simulink model "cruise"  (R2021a)
settings: Solver=VariableStepAuto  StartTime=0.0  StopTime=150.0  RelTol=1e-3
model workspace (MAT data in the model file):
  aeroCoeff.Cl0 = 0
  aeroCoeff.Cl_beta = -0.051919818
  aeroCoeff.Cl_da = -0.0981676066
  aeroCoeff.Cl_dr = 0.1746396276
  aeroCoeff.Cl_p = -0.7461562431
  aeroCoeff.Cl_r = 0.1584677463
  aeroCoeff.Cm0 = 0
  aeroCoeff.Cm_alpha = -0.208453958
  aeroCoeff.Cm_de = -3.8146754263
  aeroCoeff.Cm_q = -22.9669011845
  aeroCoeff.Cn0 = 0
  aeroCoeff.Cn_beta = 0.0540377505
  aeroCoeff.Cn_beta_dot = 0
  aeroCoeff.Cn_da = 0.0101277353
  aeroCoeff.Cn_dr = -0.4423152173
  aeroCoeff.Cn_p = -0.0208253137
  aeroCoeff.Cn_r = -0.0816662365
  aeroCoeff.Cx0 = 0
  aeroCoeff.Cx_alpha = 0.2466037589
  aeroCoeff.Cx_q = 0
  aeroCoeff.Cx_de = 0
  aeroCoeff.Cy0 = 0
  aeroCoeff.Cy_beta = -0.1443361205
  aeroCoeff.Cy_beta_dot = 0
  aeroCoeff.Cy_da = 0
  aeroCoeff.Cy_dr = 0.8693004869
  aeroCoeff.Cy_p = -0.0224336303
  aeroCoeff.Cy_r = 0.1468814604
  aeroCoeff.Cz0 = -0.5167063636
  aeroCoeff.Cz_alpha = -3.6783451837
  aeroCoeff.Cz_de = 0
  aeroCoeff.Cz_q = 2.429400573
  aeroCoeff.Cx_u = -0.1637449639
  aeroCoeff.Cz_u = -0.0248990234
  aeroCoeff.Cm_u = 0.0061871085
  aeroCoeff.Cx_alpha_dot = 0
  aeroCoeff.Cz_alpha_dot = -3.5068180832
  aeroCoeff.Cm_alpha_dot = -9.6904377913
  aeroCoeff.CL = 0.515838963283
  asymmSys.P = [-3.42306054866  0  0  0; 0  -0.05686151405  0  0; 0  0  -0.306843147582  0.0431305629131; 0  0  0.0431305629131  -1.21984185712]
  asymmSys.Q = [0.1443361205  -0.515838963283  0.0224336303  60.0530728646; 0  0  -1  0; 0.051919818  0  0.7461562431  -0.1584677463; -0.0540377505  0  0.0208253137  0.0816662365]
  asymmSys.R = [0  -0.8693004869; 0  0; 0.0981676066  -0.1746396276; -0.0101277353  0.4423152173]
  asymmSys.A = [-0.0421658099377  0.150695249456  -0.0065536761565  -17.5436782408; 0  0  17.5865876368  0; -0.163793657992  0  -2.44627629671  0.509567569731; 0.0385076455239  0  -0.103566365329  -0.0489311790925]
  asymmSys.B = [0  0.253954166029; 0  0; -0.32035276129  0.520769765047; -0.00302437533493  -0.344187340133]
  g = 9.80665
  initCond.x0 = [0 0 -1000]
  initCond.v0 = 72.1867618534
  initCond.euler0 = [0 0 0]
  initCond.w0 = [0 0 0]
  rho = 1.11164
  symmSys.P = [-3.42306054866  0  0  0; 0  -3.48452116909  0  0; 0  0  -0.0175260361321  0; 0  -0.169834962866  0  -14.0221567703]
  symmSys.Q = [0.1637449639  -0.2466037589  0.5167063636  0; 0.0248990234  3.6783451837  0  -197.742278103; 0  0  0  -1; -0.0061871085  0.208453958  0  22.9669011845]
  symmSys.R = [0; 0; 0; 3.8146754263]
  symmSys.A = [-0.047835836256  0.072041892159  -0.150948648514  0; -0.00714560830362  -1.05562428959  0  56.7487664754; 0  0  0  57.0579674984; 0.000527784900863  -0.00208042503405  0  -2.32523615059]
  symmSys.B = [0; 0; 0; -0.272046268544]
  vehicle.Sref = 19.8213410712
  vehicle.cbar = 1.2651477965
  vehicle.bref = 8.2092971467
  vehicle.Ixx = 8223.41527293
  vehicle.Iyy = 17849.353945
  vehicle.Izz = 32689.1284826
  vehicle.Ixz = 1155.55423289
  vehicle.m = 2722.32108207
  vehicle.Kxx = 0.04482
  vehicle.Kyy = 4.09638
  vehicle.Kzz = 0.17818
  vehicle.Kxz = 0.0063
  vehicle.mu_c = 97.6564387652
  vehicle.mu_b = 15.0499885812
  vehicle.aileron_max = 0.523598775598
  vehicle.aileron_min = -0.523598775598
  vehicle.elevator_max = 0.305432619099
  vehicle.elevator_min = -0.305432619099
  vehicle.rudder_max = 0.436332312999
  vehicle.rudder_min = -0.436332312999
libraries: pid_lib x4
settings Model: OrderedModelArguments=off  Creator=jakob  LastModifiedBy=jakob

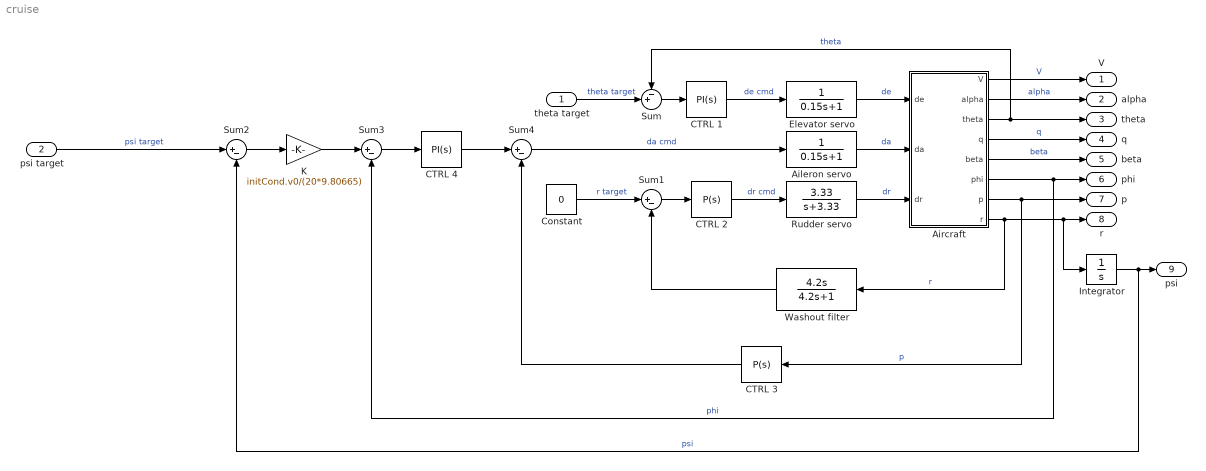
== system cruise ==
  theta target : Inport
  psi target : Inport  Port=2
  Aileron servo : TransferFcn  Denominator=[0.15 1]
  Aircraft : Subsystem
  CTRL 1 : pid_lib/PID Controller  Controller=PI  Form=Parallel  TimeDomain=Continuous-time  UseExternalTs=off  SampleTime=-1  IntegratorMethod=Forward Euler  FilterMethod=Forward Euler  ControllerParametersSource=internal  P=-0.0959107161615802  I=-0.00101116230830857  D=0  UseFilter=on  N=100  TunerSelectOption=Transfer Function Based (PID Tuner App)  InitialConditionSource=internal  InitialConditionForIntegrator=0  InitialConditionForFilter=0  DifferentiatorICPrevScaledInput=0  ExternalReset=none  TrackingMode=off  Kt=1  LimitOutput=off  SatLimitsSource=internal  UpperSaturationLimit=inf  LowerSaturationLimit=-inf  LinearizeAsGain=on  AntiWindupMode=none  Kb=1  POutMin=[]  POutMax=[]  IOutMin=[]  IOutMax=[]  DOutMin=[]  DOutMax=[]  NOutMin=[]  NOutMax=[]  SumOutMin=[]  SumOutMax=[]  SaturationOutMin=[]  SaturationOutMax=[]  PParamMin=[]  PParamMax=[]  IParamMin=[]  IParamMax=[]  DParamMin=[]  DParamMax=[]  NParamMin=[]  NParamMax=[]  KbParamMin=[]  KbParamMax=[]  KtParamMin=[]  KtParamMax=[]  KbOutMin=[]  KbOutMax=[]  KtOutMin=[]  KtOutMax=[]  IntegratorOutMin=[]  IntegratorOutMax=[]  FilterOutMin=[]  FilterOutMax=[]  SumI1OutMin=[]  SumI1OutMax=[]  SumI2OutMin=[]  SumI2OutMax=[]  SumI3OutMin=[]  SumI3OutMax=[]  SumI4OutMin=[]  SumI4OutMax=[]  SumDOutMin=[]  SumDOutMax=[]  DifferentiatorOutMin=[]  DifferentiatorOutMax=[]  FilterDiffOutCoefMin=[]  FilterDiffOutCoefMax=[]  ReciprocalOutMin=[]  ReciprocalOutMax=[]  SumDenOutMin=[]  SumDenOutMax=[]  SumNumOutMin=[]  SumNumOutMax=[]  DivideOutMin=[]  DivideOutMax=[]  UdiffTsProdOutMin=[]  UdiffTsProdOutMax=[]  NTsProdOutMin=[]  NTsProdOutMax=[]  UintegralTsProdOutMin=[]  UintegralTsProdOutMax=[]  UngainTsProdOutMin=[]  UngainTsProdOutMax=[]  IntegratorContinuousStateAttributes=''  IntegratorStateMustResolveToSignalObject=off  IntegratorRTWStateStorageClass=Auto  FilterContinuousStateAttributes=''  FilterStateMustResolveToSignalObject=off  FilterRTWStateStorageClass=Auto  ParallelPVariant=InternalParameters  IdealPVariant=Disabled  IVariant=InternalParameters  DVariant=Disabled  IntegratorVariant=Continuous  SatVariant=Disabled  AWVariant=Passthrough  PCopyVariant=Disabled  TRVariant=Disabled  FdbkBlocksVariant=Forward  IdealPFdbkVariant=Disabled  SatFdbkVariant=Disabled  DerivativeFilterVariant=Disabled  NVariant=Disabled  NCopyVariant=Disabled_SignalSpec  FilterICVariant=Disabled  IntegratorICVariant=InternalICs  ExternalResetVariant=Disabled  TRSumVariant=Passthrough  SumFdbkVariant=Disabled  SumVariant=Sum_PI  TsampFilterVariant=InternalTs  TsampNgainVariant=Passthrough  TsampIntegralVariant=Passthrough  ExternalSaturationOutDataTypeStr=Inherit: Same as second input
  CTRL 2 : pid_lib/PID Controller  Controller=P  Form=Parallel  TimeDomain=Continuous-time  UseExternalTs=off  SampleTime=-1  IntegratorMethod=Forward Euler  FilterMethod=Forward Euler  ControllerParametersSource=internal  P=-0.825543813143841  I=-0.00482340740092861  D=0  UseFilter=on  N=100  TunerSelectOption=Transfer Function Based (PID Tuner App)  InitialConditionSource=internal  InitialConditionForIntegrator=0  InitialConditionForFilter=0  DifferentiatorICPrevScaledInput=0  ExternalReset=none  TrackingMode=off  Kt=1  LimitOutput=off  SatLimitsSource=internal  UpperSaturationLimit=inf  LowerSaturationLimit=-inf  LinearizeAsGain=on  AntiWindupMode=none  Kb=1  POutMin=[]  POutMax=[]  IOutMin=[]  IOutMax=[]  DOutMin=[]  DOutMax=[]  NOutMin=[]  NOutMax=[]  SumOutMin=[]  SumOutMax=[]  SaturationOutMin=[]  SaturationOutMax=[]  PParamMin=[]  PParamMax=[]  IParamMin=[]  IParamMax=[]  DParamMin=[]  DParamMax=[]  NParamMin=[]  NParamMax=[]  KbParamMin=[]  KbParamMax=[]  KtParamMin=[]  KtParamMax=[]  KbOutMin=[]  KbOutMax=[]  KtOutMin=[]  KtOutMax=[]  IntegratorOutMin=[]  IntegratorOutMax=[]  FilterOutMin=[]  FilterOutMax=[]  SumI1OutMin=[]  SumI1OutMax=[]  SumI2OutMin=[]  SumI2OutMax=[]  SumI3OutMin=[]  SumI3OutMax=[]  SumI4OutMin=[]  SumI4OutMax=[]  SumDOutMin=[]  SumDOutMax=[]  DifferentiatorOutMin=[]  DifferentiatorOutMax=[]  FilterDiffOutCoefMin=[]  FilterDiffOutCoefMax=[]  ReciprocalOutMin=[]  ReciprocalOutMax=[]  SumDenOutMin=[]  SumDenOutMax=[]  SumNumOutMin=[]  SumNumOutMax=[]  DivideOutMin=[]  DivideOutMax=[]  UdiffTsProdOutMin=[]  UdiffTsProdOutMax=[]  NTsProdOutMin=[]  NTsProdOutMax=[]  UintegralTsProdOutMin=[]  UintegralTsProdOutMax=[]  UngainTsProdOutMin=[]  UngainTsProdOutMax=[]  IntegratorContinuousStateAttributes=''  IntegratorStateMustResolveToSignalObject=off  IntegratorRTWStateStorageClass=Auto  FilterContinuousStateAttributes=''  FilterStateMustResolveToSignalObject=off  FilterRTWStateStorageClass=Auto  ParallelPVariant=InternalParameters  IdealPVariant=Disabled  IVariant=Disabled  DVariant=Disabled  IntegratorVariant=Disabled  SatVariant=Disabled  AWVariant=Disabled  PCopyVariant=Disabled  TRVariant=Disabled  FdbkBlocksVariant=Forward  IdealPFdbkVariant=Disabled  SatFdbkVariant=Disabled  DerivativeFilterVariant=Disabled  NVariant=Disabled  NCopyVariant=Disabled_SignalSpec  FilterICVariant=Disabled  IntegratorICVariant=Disabled  ExternalResetVariant=Disabled  TRSumVariant=Passthrough  SumFdbkVariant=Disabled  SumVariant=Passthrough_P  TsampFilterVariant=InternalTs  TsampNgainVariant=Passthrough  TsampIntegralVariant=Disabled_SignalSpec  ExternalSaturationOutDataTypeStr=Inherit: Same as second input
  CTRL 3 : pid_lib/PID Controller  Controller=P  Form=Parallel  TimeDomain=Continuous-time  UseExternalTs=off  SampleTime=-1  IntegratorMethod=Forward Euler  FilterMethod=Forward Euler  ControllerParametersSource=internal  P=-2.19698599187563  I=-0.736153679717553  D=0  UseFilter=on  N=100  TunerSelectOption=Transfer Function Based (PID Tuner App)  InitialConditionSource=internal  InitialConditionForIntegrator=0  InitialConditionForFilter=0  DifferentiatorICPrevScaledInput=0  ExternalReset=none  TrackingMode=off  Kt=1  LimitOutput=off  SatLimitsSource=internal  UpperSaturationLimit=inf  LowerSaturationLimit=-inf  LinearizeAsGain=on  AntiWindupMode=none  Kb=1  POutMin=[]  POutMax=[]  IOutMin=[]  IOutMax=[]  DOutMin=[]  DOutMax=[]  NOutMin=[]  NOutMax=[]  SumOutMin=[]  SumOutMax=[]  SaturationOutMin=[]  SaturationOutMax=[]  PParamMin=[]  PParamMax=[]  IParamMin=[]  IParamMax=[]  DParamMin=[]  DParamMax=[]  NParamMin=[]  NParamMax=[]  KbParamMin=[]  KbParamMax=[]  KtParamMin=[]  KtParamMax=[]  KbOutMin=[]  KbOutMax=[]  KtOutMin=[]  KtOutMax=[]  IntegratorOutMin=[]  IntegratorOutMax=[]  FilterOutMin=[]  FilterOutMax=[]  SumI1OutMin=[]  SumI1OutMax=[]  SumI2OutMin=[]  SumI2OutMax=[]  SumI3OutMin=[]  SumI3OutMax=[]  SumI4OutMin=[]  SumI4OutMax=[]  SumDOutMin=[]  SumDOutMax=[]  DifferentiatorOutMin=[]  DifferentiatorOutMax=[]  FilterDiffOutCoefMin=[]  FilterDiffOutCoefMax=[]  ReciprocalOutMin=[]  ReciprocalOutMax=[]  SumDenOutMin=[]  SumDenOutMax=[]  SumNumOutMin=[]  SumNumOutMax=[]  DivideOutMin=[]  DivideOutMax=[]  UdiffTsProdOutMin=[]  UdiffTsProdOutMax=[]  NTsProdOutMin=[]  NTsProdOutMax=[]  UintegralTsProdOutMin=[]  UintegralTsProdOutMax=[]  UngainTsProdOutMin=[]  UngainTsProdOutMax=[]  IntegratorContinuousStateAttributes=''  IntegratorStateMustResolveToSignalObject=off  IntegratorRTWStateStorageClass=Auto  FilterContinuousStateAttributes=''  FilterStateMustResolveToSignalObject=off  FilterRTWStateStorageClass=Auto  ParallelPVariant=InternalParameters  IdealPVariant=Disabled  IVariant=Disabled  DVariant=Disabled  IntegratorVariant=Disabled  SatVariant=Disabled  AWVariant=Disabled  PCopyVariant=Disabled  TRVariant=Disabled  FdbkBlocksVariant=Forward  IdealPFdbkVariant=Disabled  SatFdbkVariant=Disabled  DerivativeFilterVariant=Disabled  NVariant=Disabled  NCopyVariant=Disabled_SignalSpec  FilterICVariant=Disabled  IntegratorICVariant=Disabled  ExternalResetVariant=Disabled  TRSumVariant=Passthrough  SumFdbkVariant=Disabled  SumVariant=Passthrough_P  TsampFilterVariant=InternalTs  TsampNgainVariant=Passthrough  TsampIntegralVariant=Disabled_SignalSpec  ExternalSaturationOutDataTypeStr=Inherit: Same as second input
  CTRL 4 : pid_lib/PID Controller  Controller=PI  Form=Parallel  TimeDomain=Continuous-time  UseExternalTs=off  SampleTime=-1  IntegratorMethod=Forward Euler  FilterMethod=Forward Euler  ControllerParametersSource=internal  P=-1.66466876697902  I=-0.145963586127284  D=-0.21492256580816  UseFilter=on  N=177.754765767358  TunerSelectOption=Transfer Function Based (PID Tuner App)  InitialConditionSource=internal  InitialConditionForIntegrator=0  InitialConditionForFilter=0  DifferentiatorICPrevScaledInput=0  ExternalReset=none  TrackingMode=off  Kt=1  LimitOutput=off  SatLimitsSource=internal  UpperSaturationLimit=inf  LowerSaturationLimit=-inf  LinearizeAsGain=on  AntiWindupMode=none  Kb=1  POutMin=[]  POutMax=[]  IOutMin=[]  IOutMax=[]  DOutMin=[]  DOutMax=[]  NOutMin=[]  NOutMax=[]  SumOutMin=[]  SumOutMax=[]  SaturationOutMin=[]  SaturationOutMax=[]  PParamMin=[]  PParamMax=[]  IParamMin=[]  IParamMax=[]  DParamMin=[]  DParamMax=[]  NParamMin=[]  NParamMax=[]  KbParamMin=[]  KbParamMax=[]  KtParamMin=[]  KtParamMax=[]  KbOutMin=[]  KbOutMax=[]  KtOutMin=[]  KtOutMax=[]  IntegratorOutMin=[]  IntegratorOutMax=[]  FilterOutMin=[]  FilterOutMax=[]  SumI1OutMin=[]  SumI1OutMax=[]  SumI2OutMin=[]  SumI2OutMax=[]  SumI3OutMin=[]  SumI3OutMax=[]  SumI4OutMin=[]  SumI4OutMax=[]  SumDOutMin=[]  SumDOutMax=[]  DifferentiatorOutMin=[]  DifferentiatorOutMax=[]  FilterDiffOutCoefMin=[]  FilterDiffOutCoefMax=[]  ReciprocalOutMin=[]  ReciprocalOutMax=[]  SumDenOutMin=[]  SumDenOutMax=[]  SumNumOutMin=[]  SumNumOutMax=[]  DivideOutMin=[]  DivideOutMax=[]  UdiffTsProdOutMin=[]  UdiffTsProdOutMax=[]  NTsProdOutMin=[]  NTsProdOutMax=[]  UintegralTsProdOutMin=[]  UintegralTsProdOutMax=[]  UngainTsProdOutMin=[]  UngainTsProdOutMax=[]  IntegratorContinuousStateAttributes=''  IntegratorStateMustResolveToSignalObject=off  IntegratorRTWStateStorageClass=Auto  FilterContinuousStateAttributes=''  FilterStateMustResolveToSignalObject=off  FilterRTWStateStorageClass=Auto  ParallelPVariant=InternalParameters  IdealPVariant=Disabled  IVariant=InternalParameters  DVariant=Disabled  IntegratorVariant=Continuous  SatVariant=Disabled  AWVariant=Passthrough  PCopyVariant=Disabled  TRVariant=Disabled  FdbkBlocksVariant=Forward  IdealPFdbkVariant=Disabled  SatFdbkVariant=Disabled  DerivativeFilterVariant=Disabled  NVariant=Disabled  NCopyVariant=Disabled_SignalSpec  FilterICVariant=Disabled  IntegratorICVariant=InternalICs  ExternalResetVariant=Disabled  TRSumVariant=Passthrough  SumFdbkVariant=Disabled  SumVariant=Sum_PI  TsampFilterVariant=InternalTs  TsampNgainVariant=Passthrough  TsampIntegralVariant=Passthrough  ExternalSaturationOutDataTypeStr=Inherit: Same as second input
  Constant : Constant  Value=0
  Elevator servo : TransferFcn  Denominator=[0.15 1]
  Integrator : Integrator
  K : Gain  Gain=initCond.v0/(20*9.80665)
  Rudder servo : TransferFcn  Numerator=[3.33]  Denominator=[1 3.33]
  Sum : Sum  Inputs=-+|
  Sum{1..4} (4 alike) : Sum  Inputs=|+-
  Washout filter : TransferFcn  Numerator=[4.2 0]  Denominator=[4.2 1]
  V : Outport
  alpha : Outport  Port=2
  theta : Outport  Port=3
  q : Outport  Port=4
  beta : Outport  Port=5
  phi : Outport  Port=6
  p : Outport  Port=7
  r : Outport  Port=8
  psi : Outport  Port=9
  wires:
  Aircraft/7(p) -> p/1, CTRL 3/1  "p"
  Aircraft/6(phi) -> phi/1, Sum3/2  "phi"
  Aircraft/2(alpha) -> alpha/1  "alpha"
  Aircraft/8(r) -> Integrator/1, r/1, Washout filter/1  "r"
  Aircraft/3(theta) -> Sum/1, theta/1  "theta"
  Aircraft/5(beta) -> beta/1  "beta"
  Aircraft/4(q) -> q/1  "q"
  Aircraft/1(V) -> V/1  "V"
  Sum/1 -> CTRL 1/1
  CTRL 1/1 -> Elevator servo/1  "de cmd"
  Constant/1 -> Sum1/1  "r target"
  Sum1/1 -> CTRL 2/1
  Integrator/1 -> Sum2/2, psi/1  "psi"
  Sum2/1 -> K/1
  K/1 -> Sum3/1
  Sum3/1 -> CTRL 4/1
  CTRL 4/1 -> Sum4/1
  Sum4/1 -> Aileron servo/1  "da cmd"
  CTRL 2/1 -> Rudder servo/1  "dr cmd"
  Rudder servo/1 -> Aircraft/3(dr)  "dr"
  Washout filter/1 -> Sum1/2
  CTRL 3/1 -> Sum4/2
  Elevator servo/1 -> Aircraft/1(de)  "de"
  theta target/1 -> Sum/2  "theta target"
  Aileron servo/1 -> Aircraft/2(da)  "da"
  psi target/1 -> Sum2/1  "psi target"

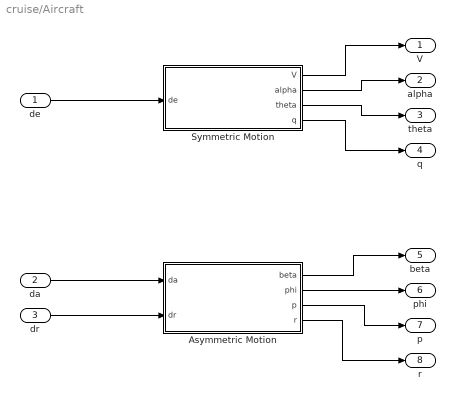
== system cruise/Aircraft ==
  de : Inport
  da : Inport  Port=2
  dr : Inport  Port=3
  Asymmetric Motion : Subsystem
  Symmetric Motion : Subsystem
  V : Outport
  alpha : Outport  Port=2
  theta : Outport  Port=3
  q : Outport  Port=4
  beta : Outport  Port=5
  phi : Outport  Port=6
  p : Outport  Port=7
  r : Outport  Port=8
  wires:
  Asymmetric Motion/2(phi) -> phi/1
  Symmetric Motion/1(V) -> V/1
  dr/1 -> Asymmetric Motion/2(dr)
  Asymmetric Motion/1(beta) -> beta/1
  Symmetric Motion/3(theta) -> theta/1
  Symmetric Motion/4(q) -> q/1
  Asymmetric Motion/4(r) -> r/1
  Asymmetric Motion/3(p) -> p/1
  Symmetric Motion/2(alpha) -> alpha/1
  da/1 -> Asymmetric Motion/1(da)
  de/1 -> Symmetric Motion/1(de)

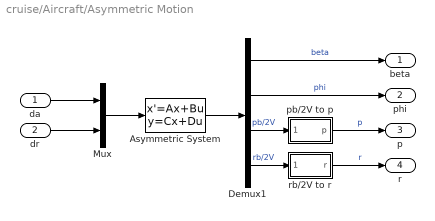
== system cruise/Aircraft/Asymmetric Motion ==
  da : Inport
  dr : Inport  Port=2
  Asymmetric System : StateSpace  A=asymmSys.A  B=asymmSys.B  C=eye(4)  D=zeros(4,2)  InitialCondition=zeros(4,1)
  Demux1 : Demux
  Mux : Mux  Inputs=2
  pb/2V to p : Subsystem
  rb/2V to r : Subsystem
  beta : Outport
  phi : Outport  Port=2
  p : Outport  Port=3
  r : Outport  Port=4
  wires:
  Mux/1 -> Asymmetric System/1
  Demux1/3 -> pb/2V to p/1(pb/2V)  "pb/2V"
  Demux1/4 -> rb/2V to r/1(rb/2V)  "rb/2V"
  rb/2V to r/1(r) -> r/1  "r"
  Asymmetric System/1 -> Demux1/1
  pb/2V to p/1(p) -> p/1  "p"
  Demux1/1 -> beta/1  "beta"
  Demux1/2 -> phi/1  "phi"
  dr/1 -> Mux/2
  da/1 -> Mux/1

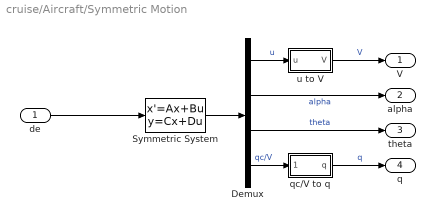
== system cruise/Aircraft/Symmetric Motion ==
  de : Inport
  Demux : Demux
  Symmetric System : StateSpace  A=symmSys.A  B=symmSys.B  C=eye(4)  D=zeros(4,1)  InitialCondition=zeros(4, 1)
  qc/V to q : Subsystem
  u to V : Subsystem
  V : Outport
  alpha : Outport  Port=2
  theta : Outport  Port=3
  q : Outport  Port=4
  wires:
  Demux/4 -> qc/V to q/1(qc/V)  "qc/V"
  Symmetric System/1 -> Demux/1
  qc/V to q/1(q) -> q/1  "q"
  u to V/1(V) -> V/1  "V"
  de/1 -> Symmetric System/1
  Demux/1 -> u to V/1(u)  "u"
  Demux/3 -> theta/1  "theta"
  Demux/2 -> alpha/1  "alpha"

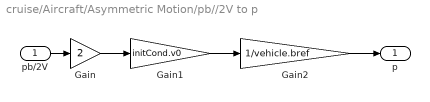
== system cruise/Aircraft/Asymmetric Motion/pb//2V to p ==
  pb/2V : Inport
  Gain : Gain  Gain=2
  Gain1 : Gain  Gain=initCond.v0
  Gain2 : Gain  Gain=1/vehicle.bref
  p : Outport
  wires:
  Gain/1 -> Gain1/1
  Gain1/1 -> Gain2/1
  pb/2V/1 -> Gain/1
  Gain2/1 -> p/1

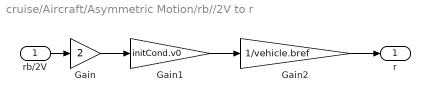
== system cruise/Aircraft/Asymmetric Motion/rb//2V to r ==
  rb/2V : Inport
  Gain : Gain  Gain=2
  Gain1 : Gain  Gain=initCond.v0
  Gain2 : Gain  Gain=1/vehicle.bref
  r : Outport
  wires:
  Gain/1 -> Gain1/1
  Gain1/1 -> Gain2/1
  rb/2V/1 -> Gain/1
  Gain2/1 -> r/1

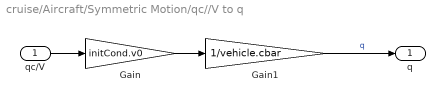
== system cruise/Aircraft/Symmetric Motion/qc//V to q ==
  qc/V : Inport
  Gain : Gain  Gain=initCond.v0
  Gain1 : Gain  Gain=1/vehicle.cbar
  q : Outport
  wires:
  Gain/1 -> Gain1/1
  Gain1/1 -> q/1  "q"
  qc/V/1 -> Gain/1

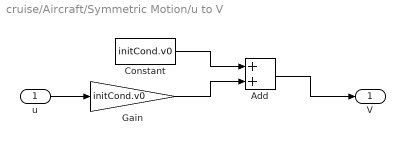
== system cruise/Aircraft/Symmetric Motion/u to V ==
  u : Inport
  Add : Sum
  Constant : Constant  Value=initCond.v0
  Gain : Gain  Gain=initCond.v0
  V : Outport
  wires:
  Gain/1 -> Add/2
  u/1 -> Gain/1
  Constant/1 -> Add/1
  Add/1 -> V/1
